simulink model "ACGen_DCLink"  (R2019b)
settings: Solver=ode3  StartTime=0.0  StopTime=0.6  FixedStep=Ts  RelTol=1e-3  EnableMultiTasking=on
PreLoadFcn:
  | warning off Simulink:Commands:LoadMdlParameterizedLink
  | Ts=1e-5;
PostLoadFcn:
  | warning off Simulink:Commands:LoadMdlParameterizedLink
  | warning off Simulink:Engine:UsingDiscreteSolver
libraries: powerlib x3, Generator_Lib x1, simulink x1
Description:
  | Copyright 2014-2019 The MathWorks, Inc.
settings Model: Creator=smiller  LastModifiedBy=smiller
settings DataIOCC: LimitDataPoints=on  SaveFormat=Array  ReturnWorkspaceOutputs=off
settings OptimizationCC: LifeSpan=inf
settings DebuggingCC: UnderspecifiedInitializationDetection=Classic  MergeDetectMultiDrivingBlocksExec=none  SolverPrmCheckMsg=warning  AllowSymbolicDim=off  StateNameClashWarn=warning  PregeneratedLibrarySubsystemCodeDiagnostic=none  SFUnexpectedBacktrackingDiag=warning  SFNoUnconditionalDefaultTransitionDiag=warning  SFExecutionAtInitializationDiag=none  ArithmeticOperatorsInVariantConditions=warning
settings HardwareCC: ProdBitPerPointer=32  ProdBitPerSizeT=32  ProdBitPerPtrDiffT=32  ProdLargestAtomicFloat=None  ProdIntDivRoundTo=Undefined  ProdEndianess=Unspecified  ProdWordSize=32  ProdHWDeviceType=32-bit Generic
settings ModelReferenceCC: PropagateSignalLabelsOutOfModel=off
settings SFSimCC: SimUseLocalCustomCode=off  CustomCodeUndefinedFunction=UseInterfaceOnly
settings RTWCC: RTWUseLocalCustomCode=off
settings CodeAppCC: StateflowObjectComments=on
settings GRTTargetCC: TargetLangStandard=C89/C90 (ANSI)  GeneratePreprocessorConditionals=Disable all
settings ConfigComp: CovMetricSettings=dw  CovHtmlReporting=on  CovSaveCumulativeToWorkspaceVar=on  CovSaveSingleToWorkspaceVar=on  CovExternalEMLEnable=off  CovSFcnEnable=off
settings SimscapeCC: SimscapeNormalizeSystem=off  SimscapeNominalValues="[{\"value\":\"10\",\"unit\":\"V\"},{\"value\":\"1\",\"unit\":\"A\"},{\"value\":\"10\",\"unit\":\"N*m\"},{\"value\":\"10\",\"unit\":\"bar\"},{\"value\":\"100\",\"unit\":\"kJ/kg\"},{\"value\":\"1\",\"unit\":\"kW\"},{\"value\":\"300\",\"unit\":\"K\"},{\"value\":\"100\",\"unit\":\"cm^3/s\"},{\"value\":\"1\",\"unit\":\"kN\"},{\"value\":\"1\",\"unit\":\"g/cm^3\"},{\"value\":\"1\",\"unit\":\"l\"},{\"value\":\"1\",\"unit\":\"cm^2\"},{\"value\":\"60\",\"unit\":\"Hz\"}]"

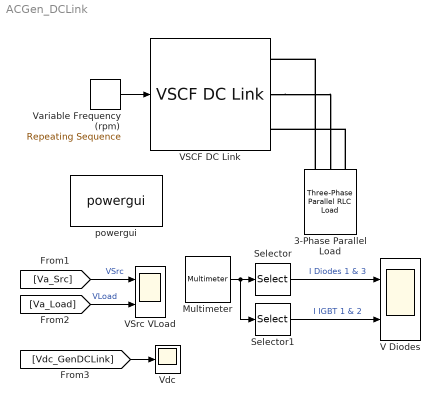
== system ACGen_DCLink ==
  3-Phase Parallel Load : powerlib/Elements/Three-Phase Parallel RLC Load  LConnTagsString=A|B|C  Configuration=Y (grounded)  NominalVoltage=200  Vabc=[1e3 1e3 1e3]  Vabcp=[1e3 1e3 1e3]  NominalFrequency=400  UnbalancedPower=off  ActivePower=50e3  InductivePower=0  CapacitivePower=0  Pabc=[10e3 9e3 11e3]  QLabc=[100 90 110]  QCabc=[100 90 110]  Pabcp=[10e3 9e3 11e3]  QLabcp=[100 90 110]  QCabcp=[100 90 110]  Measurements=None  LoadType=constant Z
      settings: SourceProductName=Simscape Electrical
  Multimeter : powerlib/Measurements/Multimeter  Tag=PoWeRsYsTeMmEaSuReMeNt  PhasorSimulation=off  OutputType=Magnitude  sel=[1 3 7 8]  L=12  Gain=[1 1 1 1]  yselected="{'Isw1: VSCF DC Link/Rect and Inv/Rectifier','Isw3: VSCF DC Link/Rect and Inv/Rectifier','Isw1: VSCF DC Link/Rect and Inv/PWM  IGBT Inverter','Isw2: VSCF DC Link/Rect and Inv/PWM  IGBT Inverter'};"  PSBOutputType=1  PSBequivalent=0  AxesSetting=[0,0.1,-100,100]  Display=0  SavedBlockNames=-11
      settings: AttributesFormatString=\n  SourceProductName=Simscape Electrical
  Selector : Selector  InputPortWidth=4  IndexOptions=Index vector (dialog)  Indices=[1 2]  OutputSizes=1
  Selector1 : Selector  InputPortWidth=4  IndexOptions=Index vector (dialog)  Indices=[3 4]  OutputSizes=1
  V Diodes : Scope  NumInputPorts=2
  VSCF DC Link : Generator_Lib/Generator/VSCF DC Link  VariantControl=VSCF_DC_Link  GenTypeDCLink=Ideal
      link override DC Link Gen: BlockChoice=Ideal
      link override DC Link Gen/Sync Mach/Simplified Synchronous Machine SI Units/Electrical model: BlockChoice=Discrete
      link override DC Link Gen/Sync Mach/Simplified Synchronous Machine SI Units/From: GotoTag=tpd1310825_afd0_45f3_9514_ec394a16d076
      link override DC Link Gen/Sync Mach/Simplified Synchronous Machine SI Units/Goto: GotoTag=tpf776af48_5bc0_4b5a_a6c9_b38312d96eab
      link override DC Link Gen/Sync Mach/Simplified Synchronous Machine SI Units/Mechanical model: BlockChoice=Discrete w input
      mask Display:
      | image(imread('Gen_VSCF_DCLink_IMAGE.JPG','jpg'))
      | port_label('RConn',1,'A');
      | port_label('RConn',2,'B');
      | port_label('RConn',3,'C');
      | port_label('Input',1,'Spd');
  VSrc VLoad : Scope  NumInputPorts=2
  Variable Frequency (rpm) : simulink/Sources/Repeating Sequence  rep_seq_t=[0 1 2 3 4 5 6]/10  rep_seq_y=[1 1 0.9 0.95 0.8 0.96 1]*12000
  Vdc : Scope
  powergui : powerlib/powergui  Priority=2  SimulationMode=Discrete  SampleTime=Ts  frequency=60  Iterations=50  frequencyindice=0  Pbase=100e6  ErrMax=1e-4  UnitsV=kV  UnitsW=MW  buscounter=0  FunctionMessages=off  echomessages=off  EnableUseOfTLC=off  CurrentSourceSwitches=off  DisableSnubberDevices=off  DisableRonSwitches=off  DisableVfSwitches=off  DisplayEquations=off  AutomaticDiscreteSolvers=off  SolverType=Tustin  Interpol=off  ExternalGateDelay=off  methode=off  Ts=0  x0status=blocks  SPID=off  SwTol=0  HookPort=off  NonlinearTolerance=0  nMaxIteration=15  ContinueOnMaxIteration=off  RestoreLinks=warning  ResistiveCurrentMeasurement=off  Frange=[0:2:500]  Ylog=off  Xlog=on  ShowGrid=off  save=off  variable=ZData  structure=psbbridges_str  ZoomFFT=on  StartTime=0.1-2/50  cycles=2  DisplayStyle=off  fundamental=50  FreqAxis=off  MaxFrequency=7000  frequencyindicesteady=1  RmsSteady=1  display=off
      settings: SourceProductName=Simscape Electrical
  wires:
  Variable Frequency (rpm)/1 -> VSCF DC Link/1
  [Va_Src] -> VSrc VLoad/1  "VSrc"
  [Va_Load] -> VSrc VLoad/2  "VLoad"
  Selector/1 -> V Diodes/1  "I Diodes 1 & 3"
  Selector1/1 -> V Diodes/2  "I IGBT 1 & 2"
  Multimeter/1 -> Selector/1, Selector1/1
  [Vdc_GenDCLink] -> Vdc/1
  connections:
  3-Phase Parallel Load/LConn3 -- VSCF DC Link/RConn3
  3-Phase Parallel Load/LConn1 -- VSCF DC Link/RConn1
  VSCF DC Link/RConn2 -- 3-Phase Parallel Load/LConn2
